simulink model "fuerzas_sim"  (R2014a)
settings: Solver=ode3  StartTime=0.0  StopTime=1  FixedStep=Tm  MaxStep=1e-2  RelTol=1e-3
values from neighbouring files (symbols this model uses):
  Ke = 1000    [fuerzas_var.m]    (also in hibrido_var.m)
  Kpf = (2*pi*20)^2*eye(3)    [fuerzas_var.m]    (also in hibrido_var.m)
  Kvf = 2*sqrt(Kpf)*eye(3)    [fuerzas_var.m]    (also in hibrido_var.m)
  q0 = [pi;1/4*pi]    [cartesiano_var.m]    (also in fuerzas_var.m = [0;pi/2]; hibrido_var.m = [0;pi/2])
  robotTP = robotRR    [cartesiano_var.m]    (also in fuerzas_var.m; hibrido_var.m)
undefined symbols (not defined in the file or in its folder): jacob0, modelAlpha
undefined symbols (not defined in the file): robotPlanta
libraries: roblocks x4
settings Model: Creator=Nicola  LastModifiedBy=Lucas
settings DebuggingCC: UnderspecifiedInitializationDetection=Classic  StateNameClashWarn=warning

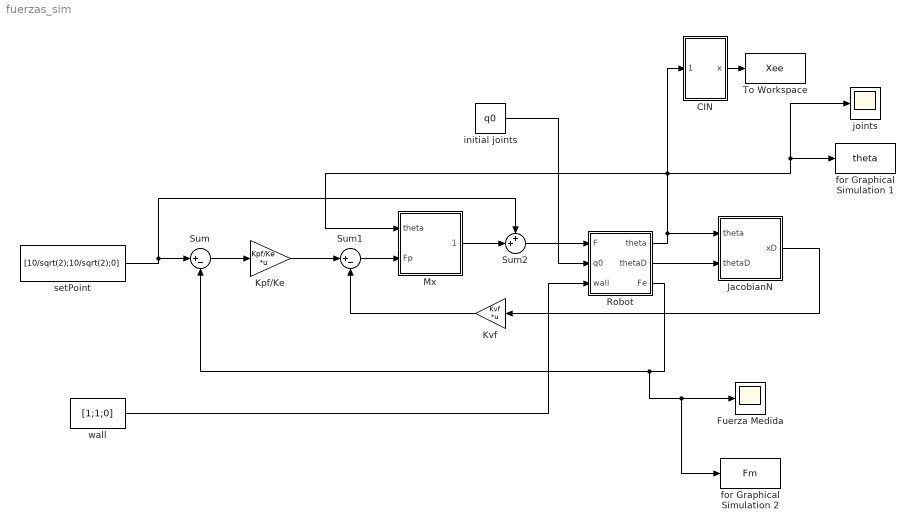
== system fuerzas_sim ==
  CIN : Subsystem
  Fuerza Medida : Scope
      settings: TimeRange=2  YMin=-1  YMax=21
  JacobianN : Subsystem
  Kpf/Ke : Gain  Gain=Kpf/Ke  Multiplication=Matrix(K*u)
  Kvf : Gain  Gain=Kvf  Multiplication=Matrix(K*u)
  Mx : Subsystem
  Robot : Subsystem
  Sum : Sum  Inputs=|+-
  Sum1 : Sum  Inputs=|+-
  Sum2 : Sum  Inputs=++|
  To Workspace : ToWorkspace  VariableName=Xee  SaveFormat=Timeseries  SampleTime=-1
  for Graphical Simulation 1 : ToWorkspace  VariableName=theta  SaveFormat=Timeseries  SampleTime=-1
  for Graphical Simulation 2 : ToWorkspace  VariableName=Fm  SaveFormat=Timeseries  SampleTime=-1
  initial joints : Constant  Value=q0
  joints : Scope
      settings: TimeRange=15  YMin=-2  YMax=3.25
  setPoint : Constant  Value=[10/sqrt(2);10/sqrt(2);0]
  wall : Constant  Value=[1;1;0]
  wires:
  initial joints/1 -> Robot/2(q0)
  Robot/1(theta) -> CIN/1(theta), joints/1, for Graphical Simulation 1/1, Mx/1(theta), JacobianN/1(theta)
  Mx/1(Mx*Fp) -> Sum2/2
  Sum1/1 -> Mx/2(Fp)
  Kvf/1 -> Sum1/2
  Sum/1 -> Kpf/Ke/1
  Kpf/Ke/1 -> Sum1/1
  JacobianN/1(xD) -> Kvf/1
  Robot/2(thetaD) -> JacobianN/2(thetaD)
  Robot/3(Fe) -> for Graphical Simulation 2/1, Fuerza Medida/1, Sum/2
  setPoint/1 -> Sum2/1, Sum/1
  wall/1 -> Robot/3(wall)
  Sum2/1 -> Robot/1(F)
  CIN/1(x) -> To Workspace/1

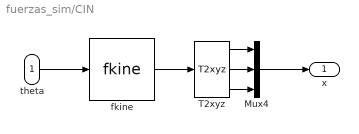
== system fuerzas_sim/CIN ==
  theta : Inport
  Mux4 : Mux  Inputs=3
  T2xyz : roblocks/Transform Conversion/T2xyz
  fkine : roblocks/Kinematics/fkine  robot=robotTP.links
  x : Outport
  wires:
  T2xyz/1 -> Mux4/1
  T2xyz/3 -> Mux4/3
  Mux4/1 -> x/1
  T2xyz/2 -> Mux4/2
  theta/1 -> fkine/1
  fkine/1 -> T2xyz/1

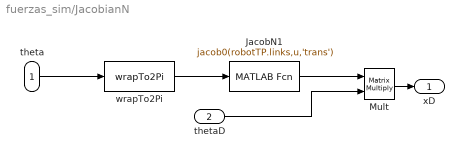
== system fuerzas_sim/JacobianN ==
  theta : Inport
  thetaD : Inport  Port=2
  JacobN1 : MATLABFcn  MATLABFcn=jacob0(robotTP.links,u,'trans')  OutputDimensions=[3,2]  Output1D=off
  Mult : Product  Multiplication=Matrix(*)
  wrapTo2Pi : MATLABFcn  MATLABFcn=wrapTo2Pi  OutputDimensions=[2,1]  Output1D=off
  xD : Outport
  wires:
  Mult/1 -> xD/1
  thetaD/1 -> Mult/2
  JacobN1/1 -> Mult/1
  wrapTo2Pi/1 -> JacobN1/1
  theta/1 -> wrapTo2Pi/1

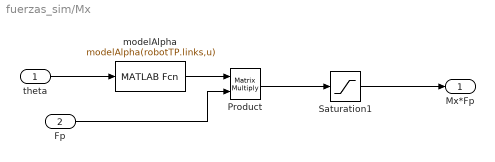
== system fuerzas_sim/Mx ==
  theta : Inport
  Fp : Inport  Port=2
  Product : Product  Multiplication=Matrix(*)
  Saturation1 : Saturate  UpperLimit=1e10  LowerLimit=-1e10
  modelAlpha : MATLABFcn  MATLABFcn=modelAlpha(robotTP.links,u)  OutputDimensions=[3,3]  Output1D=off
  Mx*Fp : Outport
  wires:
  modelAlpha/1 -> Product/1
  Fp/1 -> Product/2
  theta/1 -> modelAlpha/1
  Product/1 -> Saturation1/1
  Saturation1/1 -> Mx*Fp/1

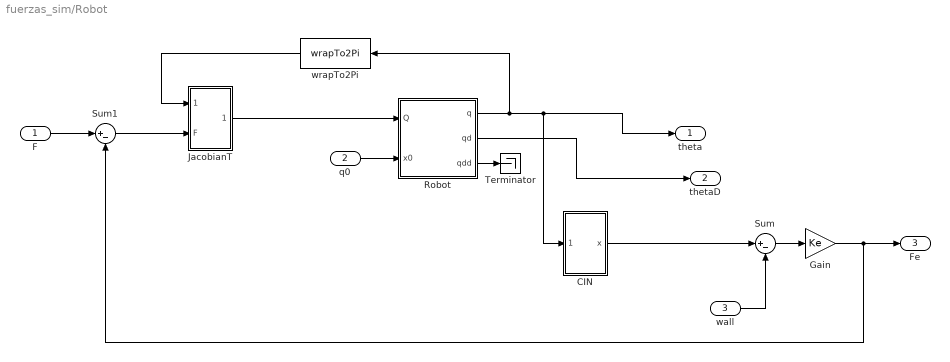
== system fuerzas_sim/Robot ==
  F : Inport
  q0 : Inport  Port=2
  wall : Inport  Port=3
  CIN : Subsystem
  Gain : Gain  Gain=Ke
  JacobianT : Subsystem
  Robot : Subsystem  AncestorBlock=roblocks/Dynamics/Robot  mask{robot=robotPlanta, q0=[0,0,0,0,0,0]}
      mask prompts: robot "Robot object"; q0 "Initial state"
      mask help: Rigid-body dynamic model of robot.
      mask init:
      | if isa(robot, 'SerialLink')
      |     rname = robot.name;
      |     %fprintf('**robot name is %s\n', rname);
      | else
      |     rname = '';
      |     n = 0
      | end
      mask Help:
      | Simulates the forward (direct) rigid-body dynamics of the robot described
      | by the given robot object.  For given applied joint torque/force it computes
      | the instaneous joint coordinates, velocities and acclerations.
      | 
      | 
      | <b>Parameters::</b>
      | 
      | robot (SerialLink) a dynamic model of an N-link serial link manipulator
      | q0 (1xN)  Initial joint coordinates
      | 
      | <b>Inputs::</b>
      | 
      | Q (1xN) the generalized joint force (torque or force) required to achieve
      | the motion state (q, qd, qdd).
      | 
      | <b>Outputs::</b>
      | 
      | q (1xN) joint coordinates
      | qd (1xN) joint coordinate velocity
      | qdd (1xN) joint coordinate acceleration
      | 
      | 
      | <b>Notes::</b>
      | 
      | - Required to simulate robot rigid body motion.
      | - Implemented using the recursive Newton-Euler scheme (RNE).
      | - A wrapper for the Toolbox method accel() which in turn depends on the
      |   method rne().
      mask Display:
      | port_label('input', 1, 'Q')
      | port_label('output', 1, 'q')
      | port_label('output', 2, 'qd')
      | port_label('output', 3, 'qdd')
      | text(0.1, 0.9,  rname, 'horizontalAlignment', 'left')
  Sum : Sum  Inputs=|+-
  Sum1 : Sum  Inputs=|+-
  Terminator : Terminator
  wrapTo2Pi : MATLABFcn  MATLABFcn=wrapTo2Pi
  theta : Outport
  thetaD : Outport  Port=2
  Fe : Outport  Port=3
  wires:
  Robot/1(q) -> wrapTo2Pi/1, CIN/1(theta), theta/1
  Robot/3(qdd) -> Terminator/1
  Robot/2(qd) -> thetaD/1
  q0/1 -> Robot/2(x0)
  JacobianT/1(tau) -> Robot/1(Q)
  wall/1 -> Sum/2
  CIN/1(x) -> Sum/1
  Sum/1 -> Gain/1
  Gain/1 -> Sum1/2, Fe/1
  Sum1/1 -> JacobianT/2(F)
  wrapTo2Pi/1 -> JacobianT/1(theta)
  F/1 -> Sum1/1

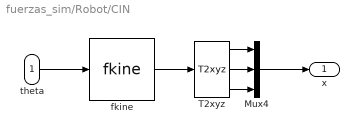
== system fuerzas_sim/Robot/CIN ==
  theta : Inport
  Mux4 : Mux  Inputs=3
  T2xyz : roblocks/Transform Conversion/T2xyz
  fkine : roblocks/Kinematics/fkine  robot=robotTP.links
  x : Outport
  wires:
  T2xyz/1 -> Mux4/1
  T2xyz/3 -> Mux4/3
  Mux4/1 -> x/1
  T2xyz/2 -> Mux4/2
  theta/1 -> fkine/1
  fkine/1 -> T2xyz/1

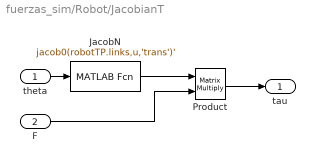
== system fuerzas_sim/Robot/JacobianT ==
  theta : Inport
  F : Inport  Port=2
  JacobN : MATLABFcn  MATLABFcn=jacob0(robotTP.links,u,'trans')'  OutputDimensions=[2,3]  Output1D=off
  Product : Product  Multiplication=Matrix(*)
  tau : Outport
  wires:
  theta/1 -> JacobN/1
  JacobN/1 -> Product/1
  F/1 -> Product/2
  Product/1 -> tau/1

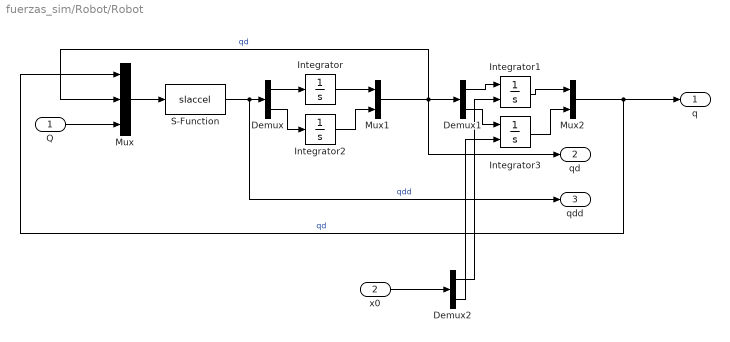
== system fuerzas_sim/Robot/Robot ==
  Q : Inport
  x0 : Inport  Port=2
  Demux : Demux  Outputs=2
  Demux1 : Demux  Outputs=2
  Demux2 : Demux  Outputs=2
  Integrator : Integrator
  Integrator1 : Integrator  InitialConditionSource=external
  Integrator2 : Integrator
  Integrator3 : Integrator  InitialConditionSource=external  InitialCondition=3/4*pi
  Mux : Mux  Inputs=3
  Mux1 : Mux  Inputs=2
  Mux2 : Mux  Inputs=2
  S-Function : S-Function  FunctionName=slaccel  Parameters=robot  EnableBusSupport=off
  q : Outport
  qd : Outport  Port=2
  qdd : Outport  Port=3
  wires:
  Q/1 -> Mux/3
  Mux/1 -> S-Function/1
  S-Function/1 -> Demux/1, qdd/1  "qdd"
  Demux/2 -> Integrator2/1
  Demux/1 -> Integrator/1
  Integrator/1 -> Mux1/1
  Integrator2/1 -> Mux1/2
  Mux1/1 -> Demux1/1, qd/1, Mux/2  "qd"
  Demux1/2 -> Integrator3/1
  Demux1/1 -> Integrator1/1
  Integrator1/1 -> Mux2/1
  Integrator3/1 -> Mux2/2
  Mux2/1 -> Mux/1, q/1  "qd"
  x0/1 -> Demux2/1
  Demux2/1 -> Integrator1/2
  Demux2/2 -> Integrator3/2
